simulink model "DETUMBLEmodel"  (R2024a)
settings: Solver=VariableStepAuto  StartTime=0.0  StopTime=16727  RelTol=1e-3
values from neighbouring files (symbols this model uses):
  I = diag([0.0046, 0.0046, 0.00145])    [BDotAlg.m]    (also in DetumbleParameters.m; bdot.m)
  Imax = 0.2143    [DetumbleParameters.m]
  Q0 = [1, 0, 0, 0]    [DetumbleParameters.m]
  w0 = [10, 10, 10]    [DetumbleParameters.m]
undefined symbols (not defined in the file or in its folder): WMM2020
libraries: matrix_library x2, simulink x1, aerolibutil x1, sharedutil x1, simulink_extras x1, aerolibgravity2 x1
settings Model: PacingRate=0.350000  Creator=dsoto  LastModifiedBy=pimpao
settings RTWCC: GPUComputeCapability=3.5

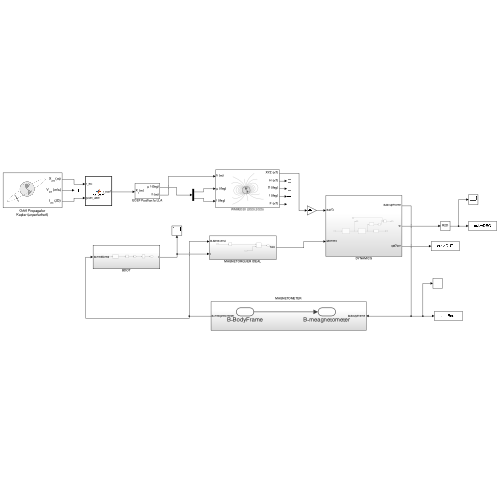
[thumbnail: Simulink's stored preview of the top-level diagram]
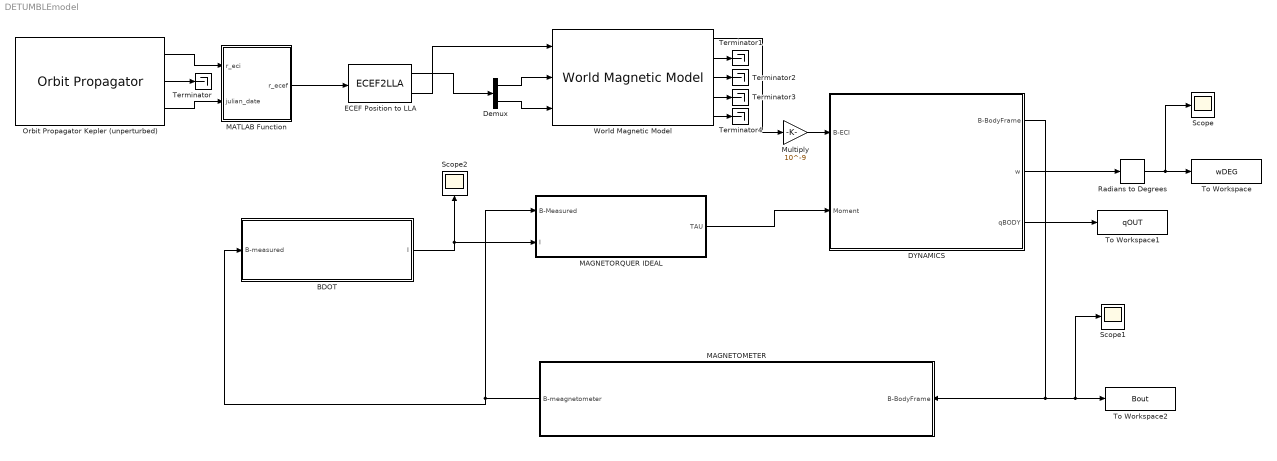
== system DETUMBLEmodel ==
  BDOT : Subsystem
  DYNAMICS : Subsystem
  Demux : Demux  Outputs=2
  ECEF Position to LLA : ECEF2LLA
  MAGNETOMETER : Subsystem
  MAGNETORQUER IDEAL : Subsystem
  MATLAB Function : MATLAB Function  TreatAsAtomicUnit=on
  Multiply : Gain  Gain=10^-9
  Orbit Propagator Kepler (unperturbed) : OrbitPropagator  semiMajorAxis=alt  eccentricity=ecc  inclination=inc  raan=raan  argPeriapsis=aop  inertialPosition=[3649700.0 3308200.0 -4676600.0]  inertialVelocity=[-2750.8 6666.4 2573.4]  fixedPosition=[-4142689.0 -2676864.7 -4669861.6]  fixedVelocity=[1452.7 -6720.7 2568.1]  customR=3396200  customMu=4.305e13  customJ2=1.0826269e-03  customOmega=4.06125949e-3
  Radians to Degrees : simulink_extras/Transformations/Radians to Degrees
  Scope : Scope
  Scope1 : Scope
  Scope2 : Scope
  Terminator{,1..4} (5 alike) : Terminator
  To Workspace : ToWorkspace  VariableName=wDEG  SaveFormat=Timeseries  SampleTime=-1
  To Workspace1 : ToWorkspace  VariableName=qOUT  SaveFormat=Timeseries  SampleTime=-1
  To Workspace2 : ToWorkspace  VariableName=Bout  SaveFormat=Timeseries  SampleTime=-1
  World Magnetic Model : aerolibgravity2/World Magnetic Model  model=WMM2020 (2020-2025)  customFile='WMM2020.COF'  units=Metric (MKS)  time_in=off  month=January  day=1  year=2020  action=Error  h_out=on  dec_out=on  inc_out=on  ti_out=on
  wires:
  DYNAMICS/1(B-BodyFrame) -> Scope1/1, To Workspace2/1, MAGNETOMETER/1(B-BodyFrame)
  MAGNETOMETER/1(B-meagnetometer) -> BDOT/1(B-measured), MAGNETORQUER IDEAL/1(B-Measured)
  BDOT/1(I) -> Scope2/1, MAGNETORQUER IDEAL/2(I)
  MAGNETORQUER IDEAL/1(TAU) -> DYNAMICS/2(Moment)
  DYNAMICS/2(w) -> Radians to Degrees/1
  Radians to Degrees/1 -> Scope/1, To Workspace/1
  DYNAMICS/3(qBODY) -> To Workspace1/1
  Multiply/1 -> DYNAMICS/1(B-ECI)
  World Magnetic Model/1 -> Multiply/1
  Orbit Propagator Kepler (unperturbed)/1 -> MATLAB Function/1(r_eci)
  Orbit Propagator Kepler (unperturbed)/2 -> Terminator/1
  MATLAB Function/1(r_ecef) -> ECEF Position to LLA/1
  ECEF Position to LLA/1 -> Demux/1
  Demux/1 -> World Magnetic Model/2
  Demux/2 -> World Magnetic Model/3
  ECEF Position to LLA/2 -> World Magnetic Model/1
  Orbit Propagator Kepler (unperturbed)/3 -> MATLAB Function/2(julian_date)
  World Magnetic Model/2 -> Terminator1/1
  World Magnetic Model/3 -> Terminator2/1
  World Magnetic Model/4 -> Terminator3/1
  World Magnetic Model/5 -> Terminator4/1

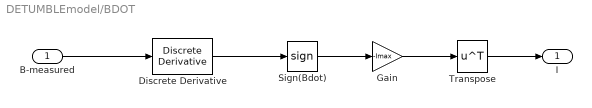
== system DETUMBLEmodel/BDOT ==
  B-measured : Inport
  Discrete Derivative : simulink/Discrete/Discrete Derivative  gainval=1.0  ICPrevScaledInput=0.0  OutMin=[]  OutMax=[]  OutDataType=fixdt(1, 16)  OutScaling=2^-10  DoSatur=off
  Gain : Gain  Gain=-Imax
  Sign(Bdot) : Signum
  Transpose : Math  Operator=transpose
  I : Outport
  wires:
  Transpose/1 -> I/1
  Discrete Derivative/1 -> Sign(Bdot)/1
  Gain/1 -> Transpose/1
  B-measured/1 -> Discrete Derivative/1
  Sign(Bdot)/1 -> Gain/1

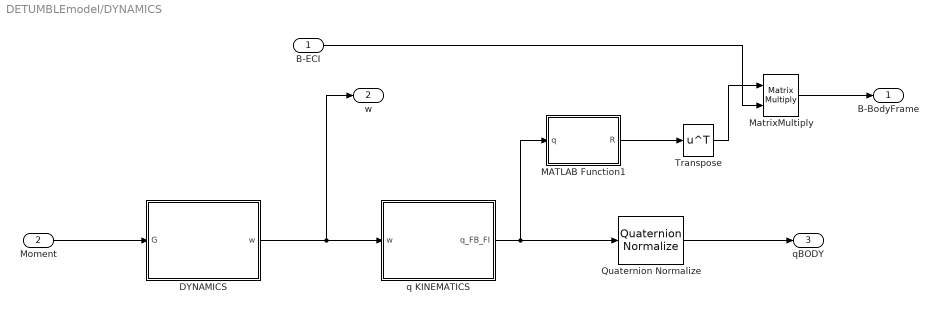
== system DETUMBLEmodel/DYNAMICS ==
  B-ECI : Inport
  Moment : Inport  Port=2
  DYNAMICS : Subsystem
  MATLAB Function1 : MATLAB Function  TreatAsAtomicUnit=on
  MatrixMultiply : Product  Multiplication=Matrix(*)
  Quaternion Normalize : sharedutil/Quaternion Normalize  aMode=aMode
  Transpose : Math  Operator=transpose
  q KINEMATICS : Subsystem
  B-BodyFrame : Outport
  w : Outport  Port=2
  qBODY : Outport  Port=3
  wires:
  Moment/1 -> DYNAMICS/1(G)
  DYNAMICS/1(w) -> w/1, q KINEMATICS/1(w)
  q KINEMATICS/1(q_FB_FI) -> MATLAB Function1/1(q), Quaternion Normalize/1
  Quaternion Normalize/1 -> qBODY/1
  MATLAB Function1/1(R) -> Transpose/1
  Transpose/1 -> MatrixMultiply/1
  B-ECI/1 -> MatrixMultiply/2
  MatrixMultiply/1 -> B-BodyFrame/1

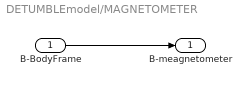
== system DETUMBLEmodel/MAGNETOMETER ==
  B-BodyFrame : Inport
  B-meagnetometer : Outport
  wires:
  B-BodyFrame/1 -> B-meagnetometer/1

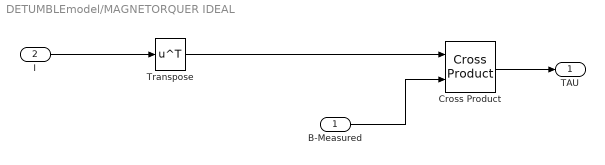
== system DETUMBLEmodel/MAGNETORQUER IDEAL ==
  B-Measured : Inport
  I : Inport  Port=2
  Cross Product : matrix_library/Cross Product
  Transpose : Math  Operator=transpose
  TAU : Outport
  wires:
  I/1 -> Transpose/1
  Transpose/1 -> Cross Product/1
  B-Measured/1 -> Cross Product/2
  Cross Product/1 -> TAU/1

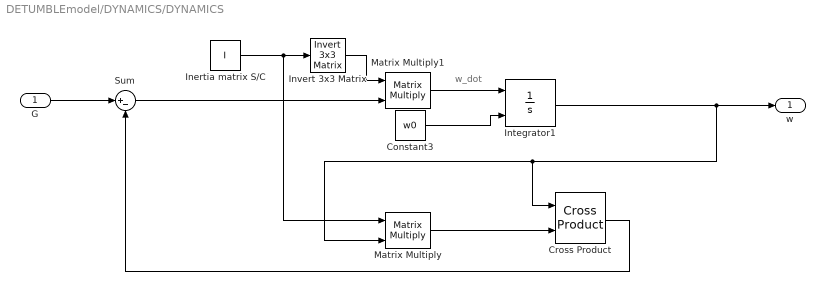
== system DETUMBLEmodel/DYNAMICS/DYNAMICS ==
  note: w_dot
  G : Inport
  Constant3 : Constant  Value=w0
  Cross Product : matrix_library/Cross Product
  Inertia matrix S/C : Constant  Value=I
  Integrator1 : Integrator  InitialConditionSource=external
  Invert 3x3 Matrix : aerolibutil/Invert  3x3 Matrix
  Matrix Multiply : Product  Multiplication=Matrix(*)
  Matrix Multiply1 : Product  Multiplication=Matrix(*)
  Sum : Sum  Inputs=|+-  OutDataTypeStr=Inherit: Same as first input
  w : Outport
  wires:
  Matrix Multiply/1 -> Cross Product/2
  Constant3/1 -> Integrator1/2
  Integrator1/1 -> Cross Product/1, Matrix Multiply/2, w/1
  Inertia matrix S/C/1 -> Matrix Multiply/1, Invert 3x3 Matrix/1
  Invert 3x3 Matrix/1 -> Matrix Multiply1/1
  Cross Product/1 -> Sum/2
  Matrix Multiply1/1 -> Integrator1/1
  G/1 -> Sum/1
  Sum/1 -> Matrix Multiply1/2

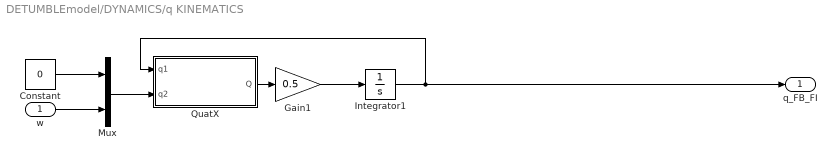
== system DETUMBLEmodel/DYNAMICS/q KINEMATICS ==
  w : Inport
  Constant : Constant  Value=0
  Gain1 : Gain  Gain=0.5
  Integrator1 : Integrator  InitialCondition=Q0
  Mux : Mux  Inputs=2
  QuatX : MATLAB Function  TreatAsAtomicUnit=on
  q_FB_FI : Outport  VectorParamsAs1DForOutWhenUnconnected=off
  wires:
  Gain1/1 -> Integrator1/1
  Integrator1/1 -> q_FB_FI/1, QuatX/1(q1)
  Mux/1 -> QuatX/2(q2)
  w/1 -> Mux/2
  Constant/1 -> Mux/1
  QuatX/1(Q) -> Gain1/1

== matlab function DETUMBLEmodel/MATLAB Function ==
  data: r_eci input; r_ecef output; julian_date input
function r_ecef = eci2ecef(r_eci, julian_date)
    % ECI to ECEF Conversion
    %
    % Inputs:
    %   r_eci       - (3x1) Vector in ECI frame
    %   julian_date - Julian date
    %
    % Output:
    %   r_ecef      - (3x1) Vector in ECEF frame

    % Constants
    JD_2000 = 2451545.0; % Julian Date of J2000.0
    sec_per_day = 86400; % Seconds per day

    % Compute the number of days from J2000.0
    days_from_J2000 = julian_date - JD_2000;

    % Compute the Greenwich Mean Sidereal Time (GMST) in seconds
    GMST_sec = 67310.54841 + (876600 * 3600 + 8640184.812866) * (days_from_J2000 / 36525) + 0.093104 * (days_from_J2000 / 36525)^2 - 6.2e-6 * (days_from_J2000 / 36525)^3;

    % Normalize GMST to be within 0 to 86400 seconds (1 day)
    GMST_sec = mod(GMST_sec, sec_per_day);

    % Convert GMST from seconds to radians
    GMST_rad = (GMST_sec / sec_per_day) * 2 * pi;

    % Rotation matrix from ECI to ECEF
    R = [cos(GMST_rad), sin(GMST_rad), 0;
         -sin(GMST_rad), cos(GMST_rad), 0;
         0, 0, 1];

    % Convert ECI coordinates to ECEF coordinates
    r_ecef = R * r_eci(:);
end

function jd = datetime2julian(utc_datetime)
    % Convert datetime to Julian Date
    %
    % Inputs:
    %   utc_datetime - [year, month, day, hour, minute, second]
    %
    % Output:
    %   jd           - Julian Date

    % Extract date and time components
    year = utc_datetime(1);
    month = utc_datetime(2);
    day = utc_datetime(3);
    hour = utc_datetime(4);
    minute = utc_datetime(5);
    second = utc_datetime(6);

    % Handle the case where month is January or February
    if month <= 2
        year = year - 1;
        month = month + 12;
    end

    % Julian Date calculation
    A = floor(year / 100);
    B = 2 - A + floor(A / 4);

    jd = floor(365.25 * (year + 4716)) + floor(30.6001 * (month + 1)) + day + B - 1524.5 + (hour + minute / 60 + second / 3600) / 24;
end

== matlab function DETUMBLEmodel/DYNAMICS/q KINEMATICS/QuatX ==
  data: q1 input; Q output; q2 input
function Q = Quat_Product(q1,q2)
% This function performs the quaternions multiplication
%
q10 = q1(1);
q1v = q1(2:4);
%
q20 = q2(1);
q2v = q2(2:4);
%
Q0 = q10*q20 - dot(q1v, q2v);
Qv = q10*q2v + q20*q1v + cross(q1v,q2v);
%
Q = [Q0;Qv];

== matlab function DETUMBLEmodel/DYNAMICS/MATLAB Function1 ==
  data: q input; R output
function R = rotation_transform(q)
    % rotation_transform - Convert quaternion to rotation matrix or apply specific rotation
    % Input:
    %   q - quaternion (4x1 vector)
    % Output:
    %   R - rotation matrix (3x3 matrix)
    
    % Ensure quaternion is normalized
    q = q / norm(q);
    
    % Quaternion components
    q0 = q(1);
    q1 = q(2);
    q2 = q(3);
    q3 = q(4);
    
    % Compute the rotation matrix
    R = [1 - 2*(q2^2 + q3^2), 2*(q1*q2 - q0*q3), 2*(q1*q3 + q0*q2);
         2*(q1*q2 + q0*q3), 1 - 2*(q1^2 + q3^2), 2*(q2*q3 - q0*q1);
         2*(q1*q3 - q0*q2), 2*(q2*q3 + q0*q1), 1 - 2*(q1^2 + q2^2)];
end
